simulink library "rgainz"  (R2022b)
settings: Solver=VariableStepAuto  StartTime=0.0  StopTime=10.0  RelTol=1e-3
undefined symbols (not defined in the file or in its folder): frameSize_samples, Fs_Hz, gain, sysin_channel_count
libraries: RgainzBtc x1
settings Model: Creator=darshana.mistry  LastModifiedBy=kl13806
settings SolverCC: AlgebraicLoopSolver=TrustRegion
settings DebuggingCC: UnconnectedInputMsg=warning  UnconnectedOutputMsg=warning  UnconnectedLineMsg=warning  SFMachineParentedDataDiag=warning  ArithmeticOperatorsInVariantConditions=warning
settings ModelReferenceCC: EnableRefExpFcnMdlSchedulingChecks=on
settings SFSimCC: CustomCodeUndefinedFunction=UseInterfaceOnly
settings RTWCC: DLArmComputeVersion=19.05

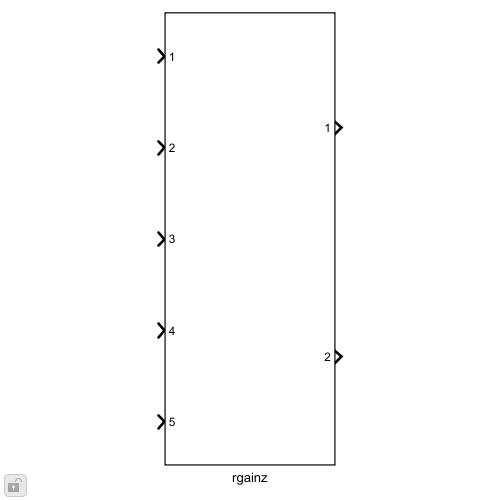
[thumbnail: Simulink's stored preview of the top-level diagram]
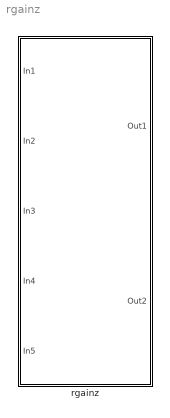
== system rgainz ==
  rgainz : Subsystem  mask(Bose Talaria RGAINZ){MaskNumRampers=sysin_channel_count, MaskInitialLinearGains=gain, nCh=sysin_channel_count, sample_rate_in_hertz=Fs_Hz, frame_size=frameSize_samples}
      mask prompts: MaskNumRampers "Number of rampers"; MaskInitialLinearGains "Initial ramper gains"; nCh "Number of Channels"
      mask init:
      | blkh = gcbh;
      | % Copy discrete mask parameters into a classdef object
      | InnerLinkConfig = RgainzConfig;
      | InnerLinkConfig.NumRampers = MaskNumRampers;
      | InnerLinkConfig.InitialLinearGains = MaskInitialLinearGains;
      | InnerLinkConfig.NumChannels = nCh;
      | InnerLinkConfig.SampleRateInHertz = sample_rate_in_hertz;
      | InnerLinkConfig.FrameSize = frame_size;

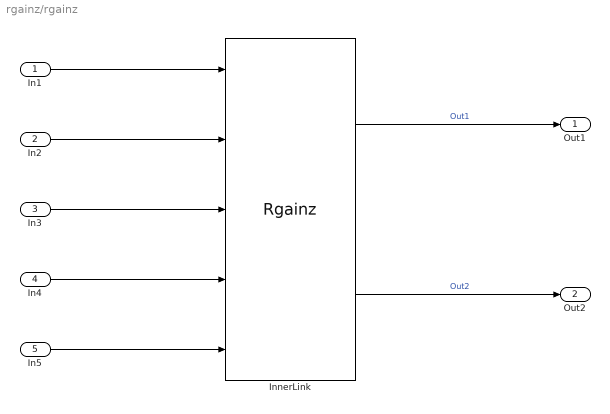
== system rgainz/rgainz ==
  In1 : Inport
  In2 : Inport  Port=2
  In3 : Inport  Port=3
  In4 : Inport  Port=4
  In5 : Inport  Port=5
  InnerLink : RgainzBtc/Rgainz  Config=InnerLinkConfig
      settings: SourceProductName=Bose Blocklib
  Out1 : Outport
  Out2 : Outport  Port=2
  wires:
  InnerLink/1 -> Out1/1  "Out1"
  InnerLink/2 -> Out2/1  "Out2"
  In1/1 -> InnerLink/1
  In2/1 -> InnerLink/2
  In3/1 -> InnerLink/3
  In4/1 -> InnerLink/4
  In5/1 -> InnerLink/5
